simulink model "Ass1"  (R2018b)
settings: Solver=VariableStepAuto  StartTime=0.0  StopTime=1220  RelTol=1e-3
values from neighbouring files (symbols this model uses):
  Bore = 82.4*10^-3    (= 0.0824)    [Car_data.m]
  Pe = P1 /(1-0.08)    [Task1.m]    (also in Task_3.m; task3solo.m)
  Stroke = 79.5*10^-3    (= 0.0795)    [Car_data.m]
  VD_e = Cyl*Vd_c    [Task1.m]    (also in Task_3.m; task3solo.m)
  w_e = 750    [Car_data.m]
libraries: qss_tb_library x10
settings Model: Creator=Mattias Langsér  LastModifiedBy=Mattias Langsér

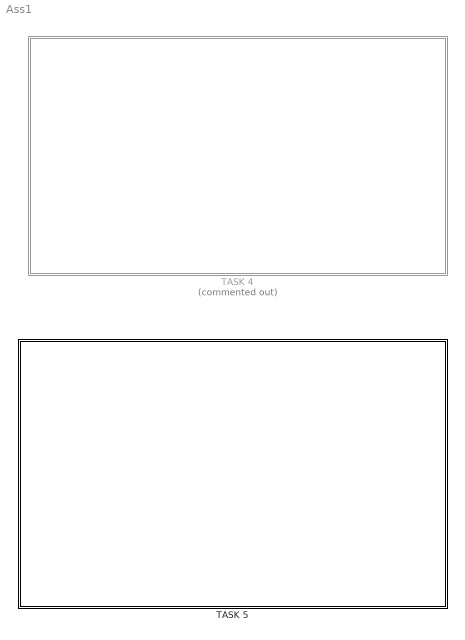
== system Ass1 ==
  "TASK 4 " : Subsystem  Commented=on
  "TASK 5 " : Subsystem

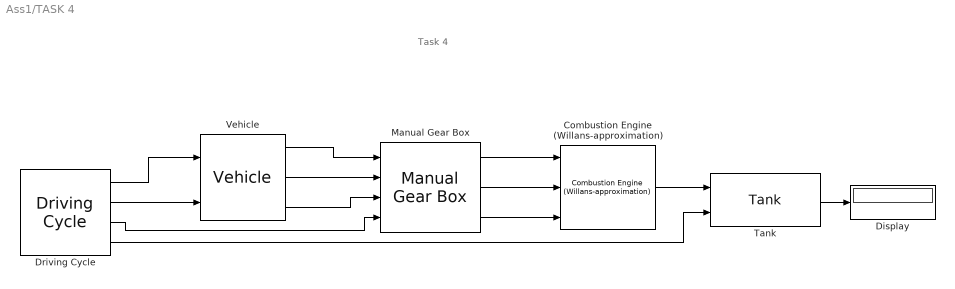
== system Ass1/TASK 4  ==
  note: Task 4
  Combustion Engine (Willans-approximation) : qss_tb_library/Energy Converter/Combustion Engine (Willans-approximation)  Tag=combustion engine  engine_type=Otto  V_d=VD_e*1000  theta_CE=J_e  S=Stroke*10^3  B=Bore*10^3  w_CE_idle=w_e*2*pi/60  P_CE_idle=P_idle  P_aux=Pe*0.08  e=Ieff_trac  PI=1  p_me0g=0.5e5  ENABLE_FUEL_CUTOFF=on  T_CE_cutoff=-5  P_CE_cutoff=0
  Display : Display
  Driving Cycle : qss_tb_library/Driving Cycle/Driving Cycle  Tag=cycle  cyclenr=Europe: NEDC manual  stepsize=1  autostop=on
  Manual Gear Box : qss_tb_library/Gear System/Manual Gear Box  Tag=transmission  i_1=G1  i_2=G2  i_3=G3  i_4=G4  i_5=G5  i_diff=1  e_GT=egb  P_GT0=P0gb  w_wheel_min=1
  Tank : qss_tb_library/Energy Source/Tank  Tag=tank  fuel=Gasoline  flag_cold_start=off
  Vehicle : qss_tb_library/Vehicle/Vehicle  Tag=vehicle  m_f=Mt  mt2m_f=Rm  A_f=Af  r_wheel=r_w  cw=cd  mu=cr
  wires:
  Driving Cycle/4 -> Tank/2
  Driving Cycle/3 -> Manual Gear Box/4
  Vehicle/2 -> Manual Gear Box/2
  Manual Gear Box/2 -> Combustion Engine (Willans-approximation)/2
  Combustion Engine (Willans-approximation)/1 -> Tank/1
  Driving Cycle/2 -> Vehicle/2
  Driving Cycle/1 -> Vehicle/1
  Manual Gear Box/1 -> Combustion Engine (Willans-approximation)/1
  Vehicle/3 -> Manual Gear Box/3
  Manual Gear Box/3 -> Combustion Engine (Willans-approximation)/3
  Vehicle/1 -> Manual Gear Box/1
  Tank/1 -> Display/1

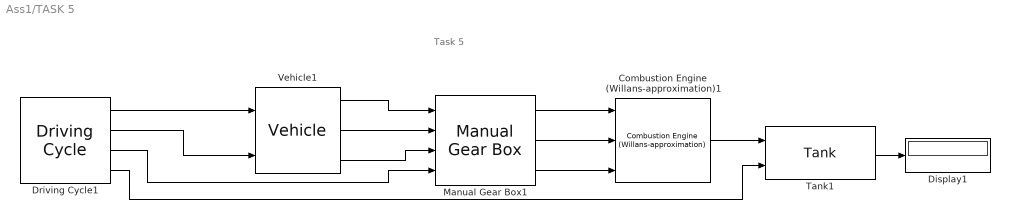
== system Ass1/TASK 5  ==
  note: Task 5
  Combustion Engine (Willans-approximation)1 : qss_tb_library/Energy Converter/Combustion Engine (Willans-approximation)  Tag=combustion engine  engine_type=Otto  V_d=VD_e*1000  theta_CE=J_e  S=Stroke*10^3  B=Bore*10^3  w_CE_idle=w_e*2*pi/60  P_CE_idle=P_idle  P_aux=Pe*0.08  e=Ieff_trac  PI=1  p_me0g=0.5e5  ENABLE_FUEL_CUTOFF=on  T_CE_cutoff=-5  P_CE_cutoff=0
  Display1 : Display
  Driving Cycle1 : qss_tb_library/Driving Cycle/Driving Cycle  Tag=cycle  cyclenr=Europe: NEDC manual  stepsize=1  autostop=on
  Manual Gear Box1 : qss_tb_library/Gear System/Manual Gear Box  Tag=transmission  i_1=G1_a  i_2=G2_a  i_3=G3_a  i_4=G4_a  i_5=G5_a  i_diff=3.77  e_GT=0.63  P_GT0=P0gb  w_wheel_min=1
  Tank1 : qss_tb_library/Energy Source/Tank  Tag=tank  fuel=Gasoline  flag_cold_start=off
  Vehicle1 : qss_tb_library/Vehicle/Vehicle  Tag=vehicle  m_f=Mt  mt2m_f=Rm  A_f=Af  r_wheel=r_w  cw=cd  mu=cr
  wires:
  Vehicle1/2 -> Manual Gear Box1/2
  Manual Gear Box1/3 -> Combustion Engine (Willans-approximation)1/3
  Combustion Engine (Willans-approximation)1/1 -> Tank1/1
  Driving Cycle1/4 -> Tank1/2
  Manual Gear Box1/2 -> Combustion Engine (Willans-approximation)1/2
  Tank1/1 -> Display1/1
  Vehicle1/3 -> Manual Gear Box1/3
  Manual Gear Box1/1 -> Combustion Engine (Willans-approximation)1/1
  Vehicle1/1 -> Manual Gear Box1/1
  Driving Cycle1/2 -> Vehicle1/2
  Driving Cycle1/3 -> Manual Gear Box1/4
  Driving Cycle1/1 -> Vehicle1/1
